simulink model "furuta_model_mabx3"  (R2023a)
settings: Solver=ode4  StartTime=0.0  StopTime=Inf  FixedStep=0.0001  RelTol=1e-3
PostLoadFcn:
  | if any(exist('dsrtsu_mdlpostloadfcn', 'file') ~= 0), dsrtsu_mdlpostloadfcn('Execute', bdroot); end
InitFcn:
  | , if any(exist('rtifpga_mdlclblib', 'file') ~= 0), rtifpga_mdlclblib('Init', bdroot); end,
  | , if any(exist('dsmpb_private', 'file') ~= 0), dsmpb_private('dsmpb_mdlclblib', 'Init', bdroot); end,
values from neighbouring files (symbols this model uses):
  N = 10    [main.m]
  nu = model.nu    [build_furuta_solver.m]    (also in furuta_model.m = 1)
  u_guess = []    [init_acados.m]    (also in main.m = u_guess.*0)
  U_max = 0.45    [build_furuta_solver.m]
  x_guess = []    [init_acados.m]    (also in main.m = x_guess.*0)
libraries: dsmpblib x7
PreSaveFcn:
  | , if any(exist('dsmpb_private', 'file') ~= 0), dsmpb_private('dsmpb_mdlclblib', 'PreSave', bdroot); end,
CloseFcn:
  | , if any(exist('dsmpb_private', 'file') ~= 0), dsmpb_private('dsmpb_mdlclblib', 'Close', bdroot); end,
settings Model: DSMPB_ID_DATA={'1',struct('BlockId','6705de95-315a-461d-bfd7-1d67e64644f6','SignalIds',{{'49302566-356f-49bf-98bb-9aa6fb4e191b','f31ab410-41a0-445c-9301-5feda3504579','b22d9c4c-e6f3-4bfe-8bb5-6e4393d82da2'}}),'2',struct('BlockId','f9af9559-7bc3-45d6-b1d0-5c923c8951f7','SignalIds',{{'640344fd-7088-4d66-828d-406be9e46a9a','f41eff98-ab4f-4f5a-b741-4dfa8486b01f','af830440-76be-4c05-a08e-eefdfbf4871e'}}),'3',struct('BlockId','0291cf52-f48d-4672-a85b-081e15b1279d','SignalIds',{{'e20d8ff1-f905-4273-8ec5-4042e75d6105'}}),'4',struct('BlockId','0211d645-065f-47f6-9582-474f3a925957','SignalIds',{{'87b883c8-a41c-4fe6-8e21-4008e8d0922c'}}),'638',struct('BlockId','b5183b78-be20-49f0-9629-cfa4d2b3c941','SignalIds',{{'6529a514-a319-41fc-97f5-7ffd89b6ed41'}}),'713',struct('BlockId','82a394dd-dc12-45ab-a2a7-927c4dc0309e','SignalIds',{{'23ea7b01-2a1b-4880-b37c-75c28e25102c'}}),'726',struct('BlockId','c77f6c66-3d30-4e59-bdfc-9087e5bcb58e','SignalIds',{{'b3d2d346-b033-4397-a923-174abd11d15c'}})}  RTICANMMDATA=struct('GeneralSetupData',struct('modelroot','C:\Users\Administrator\Furuta','generalsettings',struct('filesettings',struct('destfolder',struct('Name','RTICANMM_FILES','Check',1),'buildfolder',struct('Name','.','Check',1),'AbsDestfolder',struct('Name','C:\Users\Administrator\Furuta\RTICANMM_FILES'),'AbsBuildfolder',struct('Name','C:\Users\Administrator\Furuta'))),'options',struct('addpaths',1,'rmpaths',1,'addtrcexclusion',false,'cannavigator',struct('checkmonitoring',0),'show_usrtrc',0,'use_usrtrc',0),'advanced',struct('options',ones(1,100)),'MPSetup',{{}},'RTI',struct('Type','DSRT','Ver','4.5','Date','02-May-2021'),'modelname','Furuta_Model','block','Furuta_Model'))  DSRTSU_INTERNAL_RTIFPGA=170  Creator=Administrator  LastModifiedBy=Administrator
settings OptimizationCC: BlockReduction=off  ConditionallyExecuteInputs=off  OptimizeBlockIOStorage=off  BufferReuse=off
settings DebuggingCC: TasksWithSamePriorityMsg=none
settings HardwareCC: ProdBitPerPointer=32  ProdBitPerSizeT=32  ProdBitPerPtrDiffT=32  ProdLargestAtomicInteger=Integer  ProdWordSize=32  ProdLongLongMode=on  ProdHWDeviceType=Custom Processor->Custom
settings ModelReferenceCC: EnableParallelModelReferenceBuilds=on
settings RTWCC: Description=dSPACE Run-Time Target (for VEOS on Windows and ConfigurationDesk)  SystemTargetFile=dsrt.tlc  GenCodeOnly=on  MakeCommand=make_dsrt  TemplateMakefile=dsrt_default_tmf  RTWVerbose=off
settings RTWCC: CustomInclude=|
  | "C:\Users\Administrator\acados_neu\buildDS1403\install\include"
  | "C:\Users\Administrator\acados_neu\buildDS1403\install\include\blasfeo"
  | "C:\Users\Administrator\acados_neu\buildDS1403\install\include\blasfeo\include"
  | "C:\Users\Administrator\acados_neu\buildDS1403\install\include\acados_c"
  | "C:\Users\Administrator\acados_neu\buildDS1403\install\include\hpipm"
  | "C:\Users\Administrator\acados_neu\buildDS1403\install\include\hpipm\include"
  | "C:\Users\Administrator\acados_neu\buildDS1403\install\include\acados"
  | "C:\Users\Administrator\acados_neu\buildDS1403\install\include\acados\dense_qp"
  | "C:\Users\Administrator\acados_neu\buildDS1403\install\include\acados\ocp_nlp"
  | "C:\Users\Administrator\acados_neu\buildDS1403\install\include\acados\ocp_qp"
  | "C:\Users\Administrator\acados_neu\buildDS1403\install\include\acados\sim"
  | "C:\Users\Administrator\acados_neu\buildDS1403\install\include\acados\utils"
settings RTWCC: CustomSource=|
  | "C:\Users\Administrator\Furuta\c_generated_code\furuta_model\furuta_expl_ode_fun.c"
  | "C:\Users\Administrator\Furuta\c_generated_code\furuta_model\furuta_expl_ode_hess.c"
  | "C:\Users\Administrator\Furuta\c_generated_code\furuta_model\furuta_expl_vde_adj.c"
  | "C:\Users\Administrator\Furuta\c_generated_code\furuta_model\furuta_expl_vde_forw.c"
  | "C:\Users\Administrator\Furuta\c_generated_code\acados_solver_furuta.c"
settings RTWCC: CustomLibrary=|
  | "C:\Users\Administrator\acados_neu\buildDS1403\install\lib\libacados.a"
  | "C:\Users\Administrator\acados_neu\buildDS1403\install\lib\libblasfeo.a"
  | "C:\Users\Administrator\acados_neu\buildDS1403\install\lib\libhpipm.a"
settings STFCustomTargetCC: ParMdlRefBuildCompliant=on  ConcurrentExecutionCompliant=off  GRTInterface=off  UseToolchainInfoCompliant=off  SystemTargetFile=dsrt.tlc
settings GRTTargetCC: CompOptLevelCompliant=off  ConcurrentExecutionCompliant=off  CombineOutputUpdateFcns=off  MatFileLogging=off  CPPClassGenCompliant=off  UseToolchainInfoCompliant=off

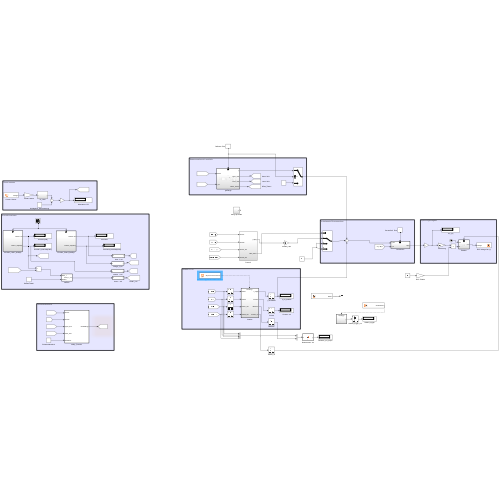
[thumbnail: Simulink's stored preview of the top-level diagram]
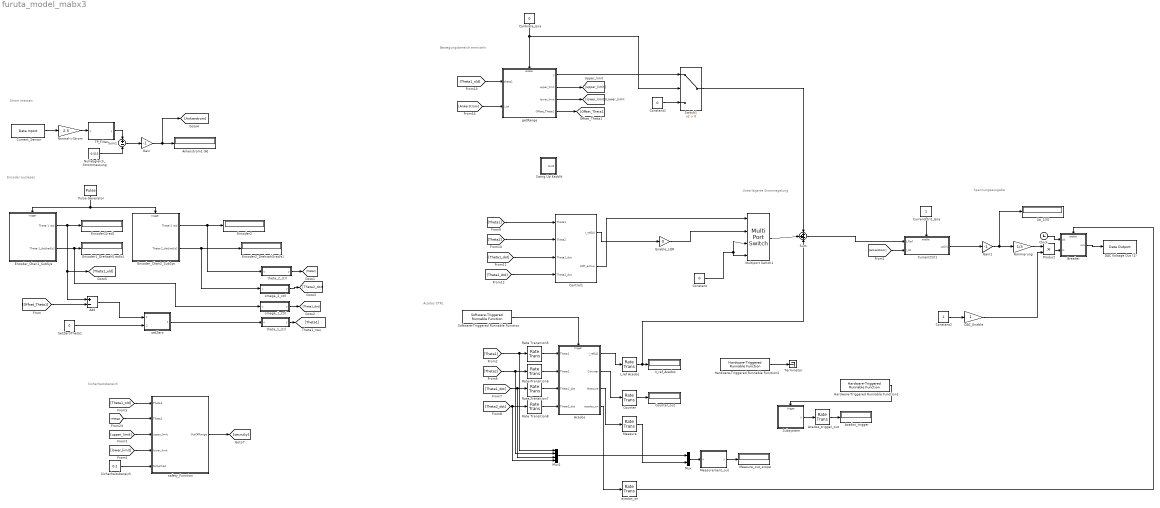
== system furuta_model_mabx3 ==
  note: Spannungsausgabe
  note: Sicherheitsbereich
  note: Bewegungsbereich ermitteln
  note: Encoder auslesen
  note: Strom messen
  note: Unterlagerte Stromregelung
  note: Acados CTRL
  Acados : Subsystem
  Acados_trigger : Display
  Acados_trigger_out : RateTransition  Deterministic=off
  Add : Sum  Inputs=+-
  Ankerstrom1 [A] : Display
  Breaker : Subsystem
  Calibrate_Ena : Constant  Value=0
  Clock : Clock
  Constant : Constant  Value=0
  Constant1 : Constant  Value=0
  Constant2 : Constant
  Control1 : Subsystem
  Counter : RateTransition  Deterministic=off
  Counter_out : Display
  CurrentCtrl1 : Subsystem
  CurrentCtrl1_Ena : Constant
  Current_Sensor : dsmpblib/Data Inport  Priority=10000
      settings: SourceProductName=dSPACE Model Interface Blockset
  DAC Voltage Out (1) : dsmpblib/Data Outport  Priority=-10000
      settings: SourceProductName=dSPACE Model Interface Blockset
  DAC_Enable : Gain
  Enable_LQR : Gain  Gain=0
  Encoder1[rad] : Display
  Encoder1_Drehzahl[rad/s] : Display
  Encoder2 : Display
  Encoder2_Drehzahl[rad/s] : Display
  Encoder_Chan1_SubSys : Subsystem
  Encoder_Chan2_SubSys : Subsystem
  Gain : Gain  Gain=-1
  Gain1 : Gain  Gain=-1
  Hardware-Triggered Runnable Function1 : dsmpblib/Hardware-Triggered Runnable Function
      settings: SourceProductName=dSPACE Model Interface Blockset
  Hardware-Triggered Runnable Function2 : dsmpblib/Hardware-Triggered Runnable Function
      settings: SourceProductName=dSPACE Model Interface Blockset
  II_ref_Acados : Display
  I_ref Acados : RateTransition  Deterministic=off
  Measure : RateTransition  Deterministic=off
  Measure_out_scope : Display
  Measurement_out : MATLAB Function  TreatAsAtomicUnit=on
  Multiport Switch1 : MultiPortSwitch  Inputs=2  DataPortForDefault=Additional data port  SaturateOnIntegerOverflow=off  InputSameDT=off
  Mux : Mux  Inputs=2
  Mux1 : Mux
  Normal->Strom : Gain  Gain=2.5
  Normierung : Gain  Gain=1/3
  Nullabgleich_Strommessung : Constant  Value=-0.015
  Product : Product
  Pulse Generator : DiscretePulseGenerator  PulseType=Time based  Period=0.001  PulseWidth=50
  Rate Transition{5..8} (4 alike) : RateTransition  Deterministic=off
  SetZeroTheta1 : Constant  Value=0
  Sicherheitsbereich : Constant  Value=0.2
  Software-Triggered Runnable Function : dsmpblib/Software-Triggered Runnable Function
      settings: SourceProductName=dSPACE Model Interface Blockset
  Subsystem : Subsystem
  Sum : Sum  Inputs=+++
  Sum1 : Sum  Inputs=+-
  Swing Up Kaddik : Subsystem
  Switch1 : Switch  Criteria=u2 > Threshold  SaturateOnIntegerOverflow=off  InputSameDT=off
  TP_Filter : Subsystem
  Terminator : Terminator
  Ua_1[V] : Display
  acados_on : RateTransition  Deterministic=off
  getRange : Subsystem
  omega_1_ctrl : MATLAB Function  TreatAsAtomicUnit=on
  omega_2_ctrl : MATLAB Function  TreatAsAtomicUnit=on
  safety_Function : MATLAB Function  TreatAsAtomicUnit=on
  setZero : MATLAB Function  TreatAsAtomicUnit=on
  theta_1_ctrl : MATLAB Function  TreatAsAtomicUnit=on
  theta_2_ctrl : MATLAB Function  TreatAsAtomicUnit=on
  wires:
  Constant1/1 -> Switch1/3
  getRange/1(y) -> Switch1/1
  [Theta1_old] -> safety_Function/1(Theta1)
  Sum/1 -> CurrentCtrl1/1(I_Ref)
  getRange/3(lower_limit) -> [lower_limit]
  Current_Sensor/1 -> Normal->Strom/1
  Pulse Generator/1 -> Encoder_Chan2_SubSys/Trigger, Encoder_Chan1_SubSys/Trigger
  Calibrate_Ena/1 -> Switch1/2, getRange/Enable
  Gain1/1 -> Normierung/1, Ua_1[V]/1
  Sum1/1 -> Gain/1
  [lower_limit] -> safety_Function/4(lower_limit)
  Gain/1 -> Ankerstrom1 [A]/1, [Ankerstrom]
  Sicherheitsbereich/1 -> safety_Function/5(Sicherheit)
  [upper_limit] -> safety_Function/3(upper_limit)
  [Ankerstrom] -> CurrentCtrl1/2(I_Ist)
  [Theta2] -> safety_Function/2(Theta2)
  TP_Filter/1(y) -> Sum1/1
  Normierung/1 -> Product/1
  [Ankerstrom] -> getRange/2(i_ist)
  CurrentCtrl1_Ena/1 -> CurrentCtrl1/Enable
  Nullabgleich_Strommessung/1 -> Sum1/2
  CurrentCtrl1/1(ua[V]) -> Gain1/1
  [Theta1_old] -> getRange/1(theta1)
  safety_Function/1(OutOfRange) -> [secruity]
  getRange/4(Offset_Theta1) -> [Offset_Theta1]
  Encoder_Chan1_SubSys/1(Theta-1 rad) -> [Theta1_old], Add/1, Encoder1[rad]/1
  getRange/2(upper_limit) -> [upper_limit]
  Normal->Strom/1 -> TP_Filter/1(u)
  [Offset_Theta1] -> Add/2
  Switch1/1 -> Sum/1
  Rate Transition5/1 -> Acados/1(Theta1)
  Acados/1(I_ref[A]) -> I_ref Acados/1
  Rate Transition8/1 -> Acados/4(Theta2_dot)
  Rate Transition7/1 -> Acados/3(Theta1_dot)
  Rate Transition6/1 -> Acados/2(Theta2)
  [Theta2] -> Mux1/2, Rate Transition6/1
  [Theta1_dot] -> Mux1/3, Rate Transition7/1
  [Theta2_dot] -> Mux1/4, Rate Transition8/1
  [Theta1] -> Control1/1(Theta1)
  [Theta2] -> Control1/2(Theta2)
  [Theta1_dot] -> Control1/3(Theta1_dot)
  [Theta2_dot] -> Control1/4(Theta2_dot)
  Control1/1(I_ref[A]) -> Enable_LQR/1
  I_ref Acados/1 -> Sum/3, II_ref_Acados/1
  Breaker/1(out) -> DAC Voltage Out (1)/1
  theta_2_ctrl/1(y) -> [Theta2]
  theta_1_ctrl/1(y) -> [Theta1]
  omega_1_ctrl/1(y) -> [Theta1_dot]
  omega_2_ctrl/1(y) -> [Theta2_dot]
  Software-Triggered Runnable Function/1 -> Acados/Trigger
  Acados/2(Counter) -> Counter/1
  Counter/1 -> Counter_out/1
  Enable_LQR/1 -> Multiport Switch1/2
  Add/1 -> setZero/1(theta_1)
  SetZeroTheta1/1 -> setZero/2(setZero)
  Control1/2(LQR_active) -> Multiport Switch1/1
  Multiport Switch1/1 -> Sum/2
  Constant/1 -> Multiport Switch1/3, Multiport Switch1/4
  [Theta1] -> Mux1/1, Rate Transition5/1
  Encoder_Chan2_SubSys/1(Theta-2 rad) -> theta_2_ctrl/1(u), Encoder2/1
  Encoder_Chan2_SubSys/2(Theta-2_dot[rad/s]) -> omega_2_ctrl/1(u), Encoder2_Drehzahl[rad/s]/1
  Encoder_Chan1_SubSys/2(Theta-1_dot[rad/s]) -> omega_1_ctrl/1(u), Encoder1_Drehzahl[rad/s]/1
  setZero/1(theta_1_out) -> theta_1_ctrl/1(u)
  Acados/3(Measure) -> Measure/1
  Measure/1 -> Mux/2
  Hardware-Triggered Runnable Function1/1 -> Subsystem/Trigger
  Subsystem/1(y) -> Acados_trigger_out/1
  Acados_trigger_out/1 -> Acados_trigger/1
  Hardware-Triggered Runnable Function2/1 -> Terminator/1
  Mux/1 -> Measurement_out/1(u)
  Mux1/1 -> Mux/1
  Measurement_out/1(y) -> Measure_out_scope/1
  Constant2/1 -> DAC_Enable/1
  DAC_Enable/1 -> Product/2
  Product/1 -> Breaker/2(in)
  Clock/1 -> Breaker/1(clk)
  Acados/4(acados_on) -> acados_on/1
  acados_on/1 -> Breaker/Enable

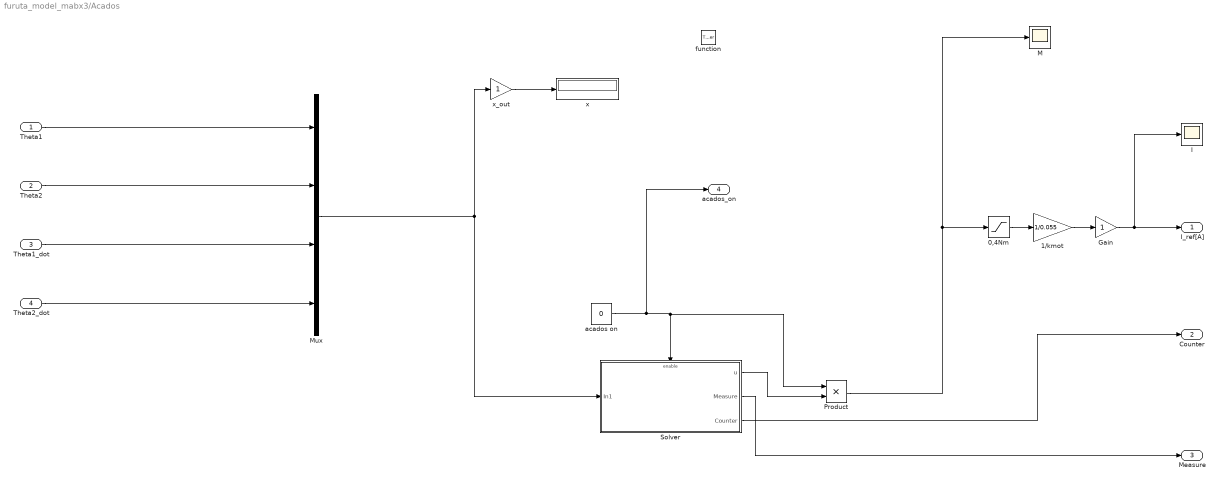
== system furuta_model_mabx3/Acados ==
  Theta1 : Inport
  Theta2 : Inport  Port=2
  Theta1_dot : Inport  Port=3
  Theta2_dot : Inport  Port=4
  function : TriggerPort  TriggerType=function-call  VariantControl=Variant
  0,4Nm : Saturate  UpperLimit=0.4  LowerLimit=-0.4
  1/kmot : Gain  Gain=1/0.055
  Gain : Gain
  I : Scope
  M : Scope
  Mux : Mux
  Product : Product
  Solver : Subsystem
  acados on : Constant  Value=0
  x : Display
  x_out : Gain
  I_ref[A] : Outport  OutputWhenDisabled=reset  InitialOutput=0  VectorParamsAs1DForOutWhenUnconnected=off
  Counter : Outport  Port=2  OutputWhenDisabled=reset  InitialOutput=0  VectorParamsAs1DForOutWhenUnconnected=off
  Measure : Outport  Port=3  OutputWhenDisabled=reset  InitialOutput=0  VectorParamsAs1DForOutWhenUnconnected=off
  acados_on : Outport  Port=4  OutputWhenDisabled=reset  InitialOutput=0  VectorParamsAs1DForOutWhenUnconnected=off
  wires:
  1/kmot/1 -> Gain/1
  Theta2/1 -> Mux/2
  Theta1/1 -> Mux/1
  0,4Nm/1 -> 1/kmot/1
  Theta2_dot/1 -> Mux/4
  Theta1_dot/1 -> Mux/3
  Gain/1 -> I/1, I_ref[A]/1
  x_out/1 -> x/1
  Mux/1 -> x_out/1, Solver/1(In1)
  Product/1 -> 0,4Nm/1, M/1
  acados on/1 -> acados_on/1, Product/1, Solver/Enable
  Solver/1(u) -> Product/2
  Solver/2(Measure) -> Measure/1
  Solver/3(Counter) -> Counter/1

== system furuta_model_mabx3/Breaker ==
  clk : Inport
  in : Inport  Port=2
  Enable : EnablePort
  MATLAB Function : MATLAB Function  TreatAsAtomicUnit=on
  out : Outport
  wires:
  MATLAB Function/1(out) -> out/1
  in/1 -> MATLAB Function/2(in)
  clk/1 -> MATLAB Function/1(clk)

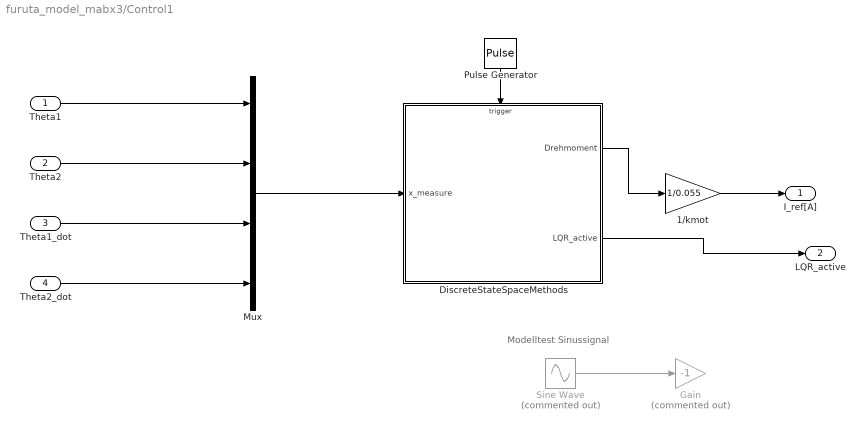
== system furuta_model_mabx3/Control1 ==
  note: Modelltest Sinussignal
  Theta1 : Inport
  Theta2 : Inport  Port=2
  Theta1_dot : Inport  Port=3
  Theta2_dot : Inport  Port=4
  1/kmot : Gain  Gain=1/0.055
  DiscreteStateSpaceMethods : Subsystem
  Gain : Gain  Commented=on  Gain=-1
  Mux : Mux
  Pulse Generator : DiscretePulseGenerator  PulseType=Time based  Period=0.001  PulseWidth=50
  Sine Wave : Sin  Commented=on  Amplitude=1.22  Bias=0.3  Frequency=0.8  SampleTime=0
  I_ref[A] : Outport  OutputWhenDisabled=reset  InitialOutput=0  VectorParamsAs1DForOutWhenUnconnected=off
  LQR_active : Outport  Port=2  OutputWhenDisabled=reset  InitialOutput=0  VectorParamsAs1DForOutWhenUnconnected=off
  wires:
  DiscreteStateSpaceMethods/1(Drehmoment) -> 1/kmot/1
  Pulse Generator/1 -> DiscreteStateSpaceMethods/Trigger
  Theta1/1 -> Mux/1
  Theta2/1 -> Mux/2
  Theta1_dot/1 -> Mux/3
  Theta2_dot/1 -> Mux/4
  Mux/1 -> DiscreteStateSpaceMethods/1(x_measure)
  Sine Wave/1 -> Gain/1
  1/kmot/1 -> I_ref[A]/1
  DiscreteStateSpaceMethods/2(LQR_active) -> LQR_active/1

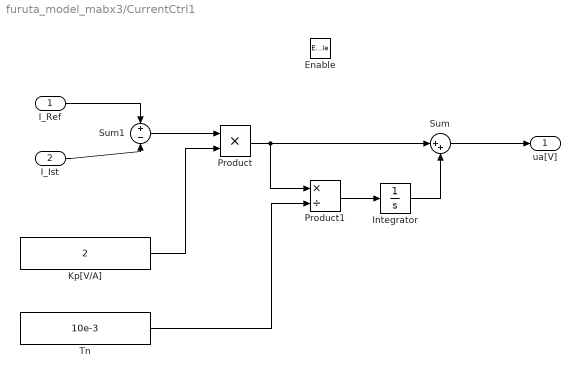
== system furuta_model_mabx3/CurrentCtrl1 ==
  I_Ref : Inport
  I_Ist : Inport  Port=2
  Enable : EnablePort  StatesWhenEnabling=reset
  Integrator : Integrator  LimitOutput=on  UpperSaturationLimit=10  LowerSaturationLimit=-10
  Kp[V/A] : Constant  Value=2
  Product : Product  RndMeth=Zero
  Product1 : Product  Inputs=*/  RndMeth=Zero
  Sum : Sum  Inputs=|++
  Sum1 : Sum  Inputs=+-
  Tn : Constant  Value=10e-3
  ua[V] : Outport  OutputWhenDisabled=reset  InitialOutput=0  VectorParamsAs1DForOutWhenUnconnected=off
  wires:
  I_Ref/1 -> Sum1/1
  I_Ist/1 -> Sum1/2
  Sum1/1 -> Product/1
  Kp[V/A]/1 -> Product/2
  Product/1 -> Sum/1, Product1/1
  Integrator/1 -> Sum/2
  Product1/1 -> Integrator/1
  Tn/1 -> Product1/2
  Sum/1 -> ua[V]/1

== system furuta_model_mabx3/Encoder_Chan1_SubSys ==
  Trigger : TriggerPort  VariantControl=(inherit)
  CONST1 : Constant  Value=pi/180*2
  DT1 : Display
  DT1 Transfer Fcn : DiscreteTransferFcn  Numerator=[50, -50]  Denominator=[1, -0.9512]
  Enc position : Display
  Enc_1 : dsmpblib/Data Inport  Priority=10000
      settings: SourceProductName=dSPACE Model Interface Blockset
  Product3 : Product  RndMeth=Zero
  Theta-1 rad : Outport  VectorParamsAs1DForOutWhenUnconnected=off
  Theta-1_dot[rad/s] : Outport  Port=2  VectorParamsAs1DForOutWhenUnconnected=off
  wires:
  Enc_1/2 -> Product3/1, Enc position/1
  CONST1/1 -> Product3/2
  DT1 Transfer Fcn/1 -> Theta-1_dot[rad/s]/1, DT1/1
  Product3/1 -> Theta-1 rad/1, DT1 Transfer Fcn/1

== system furuta_model_mabx3/Encoder_Chan2_SubSys ==
  Trigger : TriggerPort  VariantControl=(inherit)
  CONST1 : Constant  Value=pi/180*2
  DT1 Transfer Fcn : DiscreteTransferFcn  Numerator=[50, -50]  Denominator=[1, -0.9512]
  Enc_2 : dsmpblib/Data Inport  Priority=10000
      settings: SourceProductName=dSPACE Model Interface Blockset
  Product3 : Product  RndMeth=Zero
  Theta-2 rad : Outport  VectorParamsAs1DForOutWhenUnconnected=off
  Theta-2_dot[rad/s] : Outport  Port=2  VectorParamsAs1DForOutWhenUnconnected=off
  wires:
  Enc_2/2 -> Product3/1
  CONST1/1 -> Product3/2
  DT1 Transfer Fcn/1 -> Theta-2_dot[rad/s]/1
  Product3/1 -> DT1 Transfer Fcn/1, Theta-2 rad/1

== system furuta_model_mabx3/Subsystem ==
  function : TriggerPort  TriggerType=function-call  VariantControl=Variant
  MATLAB Function : MATLAB Function  TreatAsAtomicUnit=on
  y : Outport
  wires:
  MATLAB Function/1(y) -> y/1

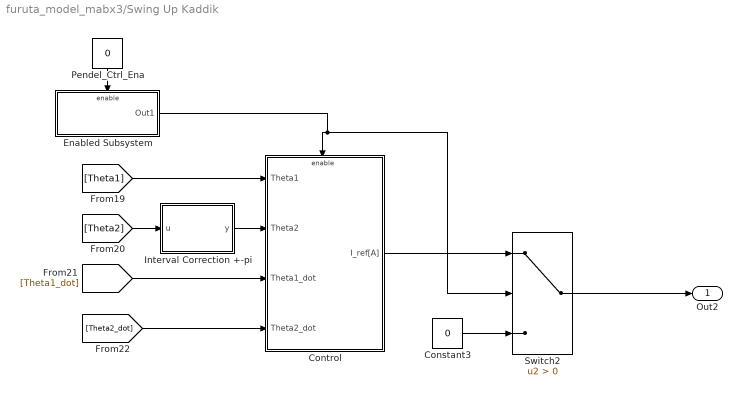
== system furuta_model_mabx3/Swing Up Kaddik ==
  Constant3 : Constant  Value=0
  Control : Subsystem
  Enabled Subsystem : Subsystem  TreatAsAtomicUnit=on
  Interval Correction +-pi : MATLAB Function  TreatAsAtomicUnit=on
  Pendel_Ctrl_Ena : Constant  Value=0
  Switch2 : Switch  Criteria=u2 > Threshold  SaturateOnIntegerOverflow=off  InputSameDT=off
  Out2 : Outport
  wires:
  Enabled Subsystem/1(Out1) -> Control/Enable, Switch2/2
  Constant3/1 -> Switch2/3
  [Theta1] -> Control/1(Theta1)
  [Theta2_dot] -> Control/4(Theta2_dot)
  [Theta1_dot] -> Control/3(Theta1_dot)
  Interval Correction +-pi/1(y) -> Control/2(Theta2)
  Control/1(I_ref[A]) -> Switch2/1
  Pendel_Ctrl_Ena/1 -> Enabled Subsystem/Enable
  [Theta2] -> Interval Correction +-pi/1(u)
  Switch2/1 -> Out2/1

== system furuta_model_mabx3/TP_Filter ==
  u : Inport
  Integrator : Integrator  UpperSaturationLimit=10  LowerSaturationLimit=-10
  Product : Product  Inputs=*/  RndMeth=Zero
  Sum1 : Sum  Inputs=+-
  ms->s : Gain  Gain=0.001
  "tau[ms}" : Constant
  y : Outport  OutputWhenDisabled=reset  InitialOutput=0  VectorParamsAs1DForOutWhenUnconnected=off
  wires:
  Integrator/1 -> y/1, Sum1/2
  "tau[ms}"/1 -> ms->s/1
  Sum1/1 -> Product/1
  u/1 -> Sum1/1
  Product/1 -> Integrator/1
  ms->s/1 -> Product/2

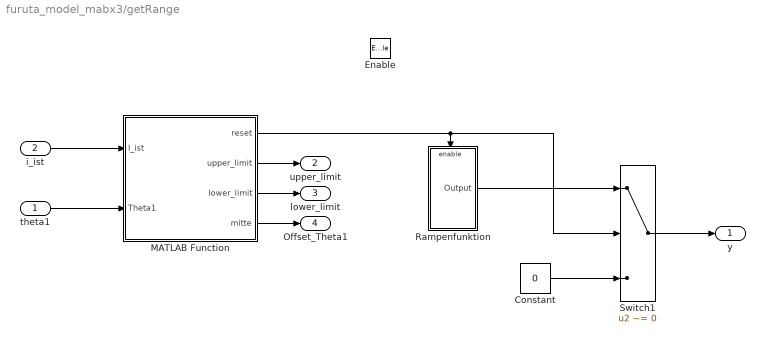
== system furuta_model_mabx3/getRange ==
  theta1 : Inport
  i_ist : Inport  Port=2
  Enable : EnablePort
  Constant : Constant  Value=0
  MATLAB Function : MATLAB Function  TreatAsAtomicUnit=on
  Rampenfunktion : Subsystem
  Switch1 : Switch  Criteria=u2 ~= 0  SaturateOnIntegerOverflow=off  InputSameDT=off
  y : Outport  OutputWhenDisabled=reset  InitialOutput=[0]
  upper_limit : Outport  Port=2
  lower_limit : Outport  Port=3
  Offset_Theta1 : Outport  Port=4
  wires:
  theta1/1 -> MATLAB Function/2(Theta1)
  i_ist/1 -> MATLAB Function/1(I_ist)
  MATLAB Function/1(reset) -> Switch1/2, Rampenfunktion/Enable
  MATLAB Function/3(lower_limit) -> lower_limit/1
  MATLAB Function/2(upper_limit) -> upper_limit/1
  Rampenfunktion/1(Output) -> Switch1/1
  Constant/1 -> Switch1/3
  Switch1/1 -> y/1
  MATLAB Function/4(mitte) -> Offset_Theta1/1

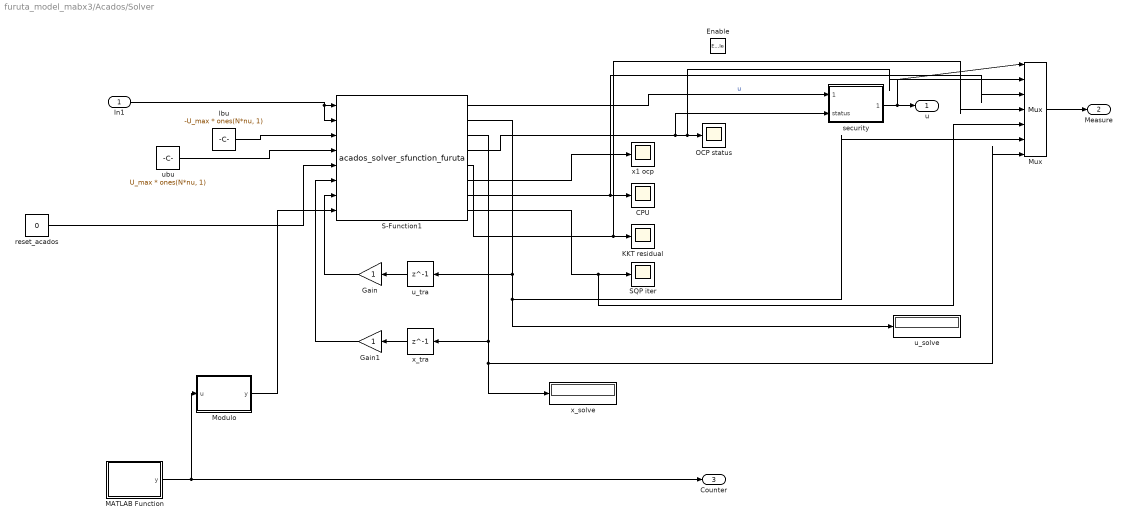
== system furuta_model_mabx3/Acados/Solver ==
  In1 : Inport
  Enable : EnablePort
  CPU : Scope
      settings: Description=status
  Gain : Gain
  Gain1 : Gain
  KKT residual : Scope
      settings: Description=status
  MATLAB Function : MATLAB Function  TreatAsAtomicUnit=on
  Modulo : MATLAB Function  TreatAsAtomicUnit=on
  Mux : Mux  Inputs=7
  OCP status : Scope
      settings: Description=status
  S-Function1 : S-Function  FunctionName=acados_solver_sfunction_furuta  SFunctionDeploymentMode=off  EnableBusSupport=off
  SQP iter : Scope
      settings: Description=status
  lbu : Constant  Value=-U_max * ones(N*nu, 1)
  reset_acados : Constant  Value=0
  security : MATLAB Function  TreatAsAtomicUnit=on
  u_solve : Display
  u_tra : Delay  DelayLength=1  InitialCondition=u_guess
  ubu : Constant  Value=U_max * ones(N*nu, 1)
  x1 ocp : Scope
      settings: Description=status
  x_solve : Display
  x_tra : Delay  DelayLength=1  InitialCondition=x_guess
  u : Outport
  Measure : Outport  Port=2
  Counter : Outport  Port=3
  wires:
  S-Function1/6 -> x1 ocp/1
  S-Function1/2 -> Mux/6, u_solve/1, u_tra/1
  In1/1 -> S-Function1/2, S-Function1/1
  S-Function1/3 -> x_tra/1, Mux/7, x_solve/1
  u_tra/1 -> Gain/1
  S-Function1/7 -> Mux/3, CPU/1
  S-Function1/5 -> Mux/4, KKT residual/1
  ubu/1 -> S-Function1/4
  lbu/1 -> S-Function1/3
  S-Function1/4 -> security/2(status), Mux/2, OCP status/1
  S-Function1/8 -> Mux/5, SQP iter/1
  S-Function1/1 -> security/1(control)  "u"
  x_tra/1 -> Gain1/1
  security/1(control_out) -> Mux/1, u/1
  Gain/1 -> S-Function1/7
  Gain1/1 -> S-Function1/6
  reset_acados/1 -> S-Function1/5
  Mux/1 -> Measure/1
  MATLAB Function/1(y) -> Modulo/1(u), Counter/1
  Modulo/1(y) -> S-Function1/8

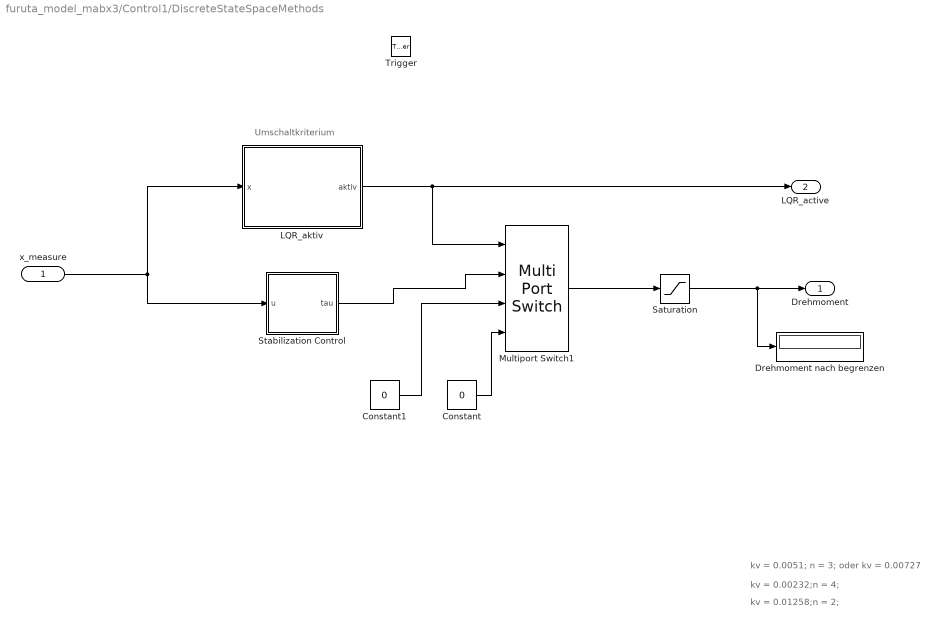
== system furuta_model_mabx3/Control1/DiscreteStateSpaceMethods ==
  note: kv = 0.00232;n = 4;
  note: kv = 0.0051; n = 3; oder kv = 0.00727
  note: Umschaltkriterium
  note: kv = 0.01258;n = 2;
  x_measure : Inport
  Trigger : TriggerPort  VariantControl=(inherit)  PortDimensions=1
  Constant : Constant  Value=0
  Constant1 : Constant  Value=0
  Drehmoment nach begrenzen : Display
  LQR_aktiv : MATLAB Function  TreatAsAtomicUnit=on
  Multiport Switch1 : MultiPortSwitch  Inputs=2  DataPortForDefault=Additional data port  SaturateOnIntegerOverflow=off  InputSameDT=off
  Saturation : Saturate  UpperLimit=0.4  LowerLimit=-0.4
  Stabilization Control : Subsystem
  Drehmoment : Outport  VectorParamsAs1DForOutWhenUnconnected=off
  LQR_active : Outport  Port=2  VectorParamsAs1DForOutWhenUnconnected=off
  wires:
  Saturation/1 -> Drehmoment nach begrenzen/1, Drehmoment/1
  LQR_aktiv/1(aktiv) -> LQR_active/1, Multiport Switch1/1
  x_measure/1 -> LQR_aktiv/1(x), Stabilization Control/1(u)
  Constant/1 -> Multiport Switch1/4
  Stabilization Control/1(tau) -> Multiport Switch1/2
  Multiport Switch1/1 -> Saturation/1
  Constant1/1 -> Multiport Switch1/3

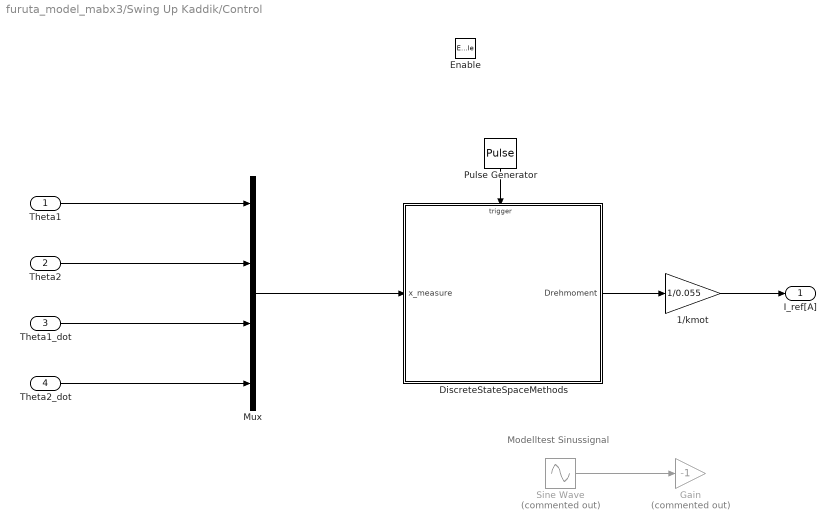
== system furuta_model_mabx3/Swing Up Kaddik/Control ==
  note: Modelltest Sinussignal
  Theta1 : Inport
  Theta2 : Inport  Port=2
  Theta1_dot : Inport  Port=3
  Theta2_dot : Inport  Port=4
  Enable : EnablePort  StatesWhenEnabling=reset
  1/kmot : Gain  Gain=1/0.055
  DiscreteStateSpaceMethods : Subsystem
  Gain : Gain  Commented=on  Gain=-1
  Mux : Mux
  Pulse Generator : DiscretePulseGenerator  PulseType=Time based  Period=0.001  PulseWidth=50
  Sine Wave : Sin  Commented=on  Amplitude=1.22  Bias=0.3  Frequency=0.8  SampleTime=0
  I_ref[A] : Outport  OutputWhenDisabled=reset  InitialOutput=0  VectorParamsAs1DForOutWhenUnconnected=off
  wires:
  DiscreteStateSpaceMethods/1(Drehmoment) -> 1/kmot/1
  Pulse Generator/1 -> DiscreteStateSpaceMethods/Trigger
  Theta1/1 -> Mux/1
  Theta2/1 -> Mux/2
  Theta1_dot/1 -> Mux/3
  Theta2_dot/1 -> Mux/4
  Mux/1 -> DiscreteStateSpaceMethods/1(x_measure)
  Sine Wave/1 -> Gain/1
  1/kmot/1 -> I_ref[A]/1

== system furuta_model_mabx3/Swing Up Kaddik/Enabled Subsystem ==
  Enable : EnablePort  StatesWhenEnabling=reset
  Pulse Generator1 : DiscretePulseGenerator  PulseType=Time based  Period=20  PulseWidth=80
  Out1 : Outport
  wires:
  Pulse Generator1/1 -> Out1/1

== system furuta_model_mabx3/getRange/Rampenfunktion ==
  Enable : EnablePort  StatesWhenEnabling=reset
  Integrator1 : Integrator  InitialCondition=0.5
  Step1 : Step  Time=0  After=0.15  SampleTime=0
  Output : Outport
  wires:
  Integrator1/1 -> Output/1
  Step1/1 -> Integrator1/1

== system furuta_model_mabx3/Control1/DiscreteStateSpaceMethods/Stabilization Control ==
  u : Inport
  Add : Sum  Inputs=++++
  Demux : Demux
  LQR_Controller : MATLAB Function  TreatAsAtomicUnit=on
  k1 : Gain  Gain=0.1
  k2 : Gain  Gain=-1.3582
  k3 : Gain  Gain=0.0544
  k4 : Gain  Gain=-0.138
  tau : Outport
  wires:
  LQR_Controller/1(drehmoment_soll) -> tau/1
  u/1 -> LQR_Controller/1(x_measure)
  Demux/1 -> k1/1
  k3/1 -> Add/3
  k2/1 -> Add/2
  Demux/4 -> k4/1
  k1/1 -> Add/1
  Demux/3 -> k3/1
  Demux/2 -> k2/1
  k4/1 -> Add/4

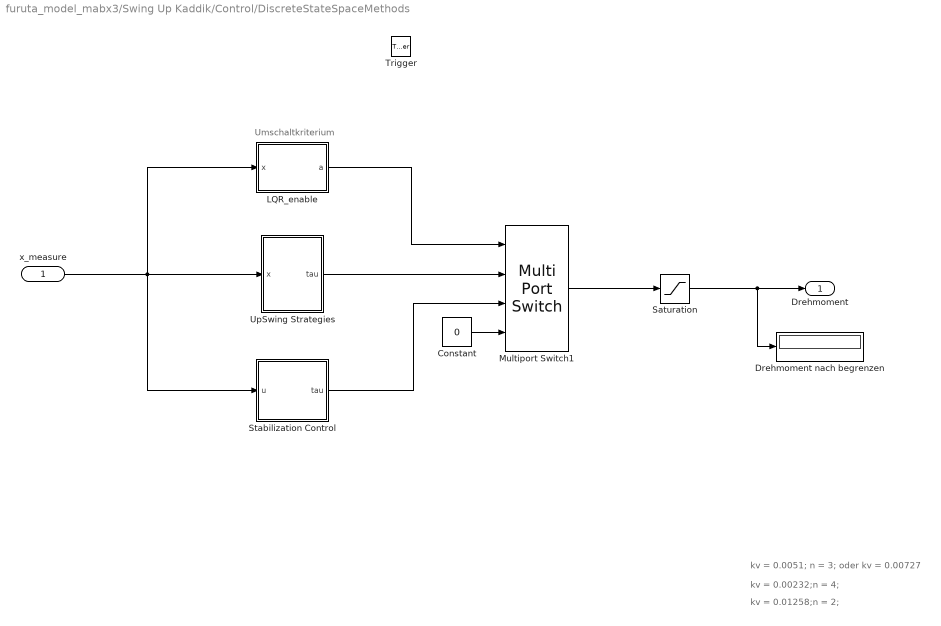
== system furuta_model_mabx3/Swing Up Kaddik/Control/DiscreteStateSpaceMethods ==
  note: kv = 0.00232;n = 4;
  note: kv = 0.0051; n = 3; oder kv = 0.00727
  note: Umschaltkriterium
  note: kv = 0.01258;n = 2;
  x_measure : Inport
  Trigger : TriggerPort  VariantControl=(inherit)  PortDimensions=1
  Constant : Constant  Value=0
  Drehmoment nach begrenzen : Display
  LQR_enable : MATLAB Function  TreatAsAtomicUnit=on
  Multiport Switch1 : MultiPortSwitch  Inputs=2  DataPortForDefault=Additional data port  SaturateOnIntegerOverflow=off  InputSameDT=off
  Saturation : Saturate  UpperLimit=0.4  LowerLimit=-0.4
  Stabilization Control : Subsystem
  UpSwing Strategies : Subsystem
  Drehmoment : Outport  VectorParamsAs1DForOutWhenUnconnected=off
  wires:
  Saturation/1 -> Drehmoment nach begrenzen/1, Drehmoment/1
  LQR_enable/1(a) -> Multiport Switch1/1
  x_measure/1 -> LQR_enable/1(x), Stabilization Control/1(u), UpSwing Strategies/1(x)
  Constant/1 -> Multiport Switch1/4
  UpSwing Strategies/1(tau) -> Multiport Switch1/2
  Stabilization Control/1(tau) -> Multiport Switch1/3
  Multiport Switch1/1 -> Saturation/1

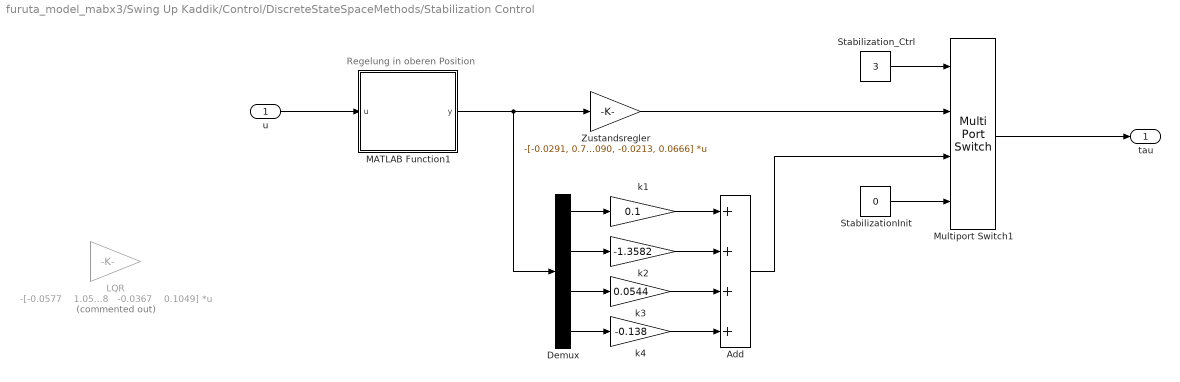
== system furuta_model_mabx3/Swing Up Kaddik/Control/DiscreteStateSpaceMethods/Stabilization Control ==
  note: Regelung in oberen Position
  u : Inport
  Add : Sum  Inputs=++++
  Demux : Demux
  LQR : Gain  Commented=on  Gain="-[-0.0577    1.0578   -0.0367    0.1049]"  Multiplication=Matrix(K*u) (u vector)
  MATLAB Function1 : MATLAB Function  TreatAsAtomicUnit=on
  Multiport Switch1 : MultiPortSwitch  Inputs=2  DataPortForDefault=Additional data port  SaturateOnIntegerOverflow=off  InputSameDT=off
  StabilizationInit : Constant  Value=0
  Stabilization_Ctrl : Constant  Value=3
  Zustandsregler : Gain  Gain=-[-0.0291, 0.7090, -0.0213, 0.0666]  Multiplication=Matrix(K*u) (u vector)
  k1 : Gain  Gain=0.1
  k2 : Gain  Gain=-1.3582
  k3 : Gain  Gain=0.0544
  k4 : Gain  Gain=-0.138
  tau : Outport
  wires:
  u/1 -> MATLAB Function1/1(u)
  StabilizationInit/1 -> Multiport Switch1/4
  Multiport Switch1/1 -> tau/1
  Add/1 -> Multiport Switch1/3
  Stabilization_Ctrl/1 -> Multiport Switch1/1
  Zustandsregler/1 -> Multiport Switch1/2
  MATLAB Function1/1(y) -> Demux/1, Zustandsregler/1
  Demux/1 -> k1/1
  k3/1 -> Add/3
  k2/1 -> Add/2
  Demux/4 -> k4/1
  k1/1 -> Add/1
  Demux/3 -> k3/1
  Demux/2 -> k2/1
  k4/1 -> Add/4

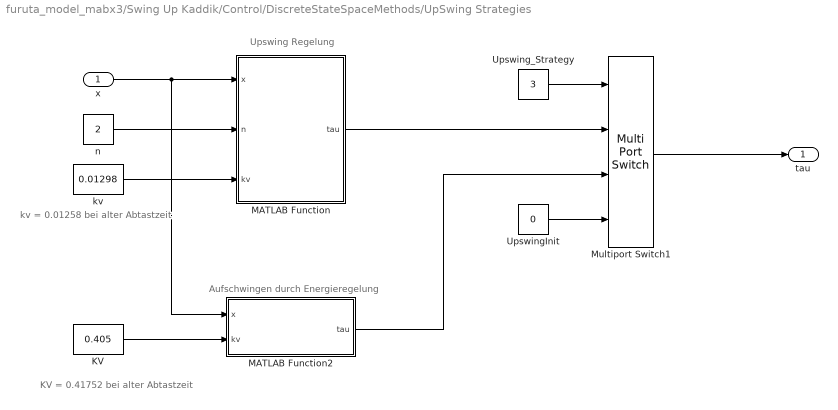
== system furuta_model_mabx3/Swing Up Kaddik/Control/DiscreteStateSpaceMethods/UpSwing Strategies ==
  note: kv = 0.01258 bei alter Abtastzeit
  note: KV = 0.41752 bei alter Abtastzeit
  note: Upswing Regelung
  note: Aufschwingen durch Energieregelung
  x : Inport
  KV : Constant  Value=0.405
  MATLAB Function : MATLAB Function  TreatAsAtomicUnit=on
  MATLAB Function2 : MATLAB Function  TreatAsAtomicUnit=on
  Multiport Switch1 : MultiPortSwitch  Inputs=2  DataPortForDefault=Additional data port  SaturateOnIntegerOverflow=off  InputSameDT=off
  UpswingInit : Constant  Value=0
  Upswing_Strategy : Constant  Value=3
  kv : Constant  Value=0.01298
  n : Constant  Value=2
  tau : Outport
  wires:
  x/1 -> MATLAB Function/1(x), MATLAB Function2/1(x)
  kv/1 -> MATLAB Function/3(kv)
  MATLAB Function/1(tau) -> Multiport Switch1/2
  n/1 -> MATLAB Function/2(n)
  KV/1 -> MATLAB Function2/2(kv)
  Upswing_Strategy/1 -> Multiport Switch1/1
  MATLAB Function2/1(tau) -> Multiport Switch1/3
  Multiport Switch1/1 -> tau/1
  UpswingInit/1 -> Multiport Switch1/4

== matlab function furuta_model_mabx3/Acados/Solver/MATLAB Function ==
  data: y output
function y = fcn()
%#codegen

persistent zahl
if isempty(zahl)
    zahl=0;
else
    zahl=zahl+1;
end
y = zahl;

== matlab function furuta_model_mabx3/setZero ==
  data: theta_1 input; theta_1_out output; setZero input
function theta_1_out = fcn(theta_1,setZero)
%#codegen
persistent offset

theta_1_out=theta_1;

if setZero==1 && isempty(offset)
    offset = theta_1;
end
if ~isempty(offset)
    theta_1_out = theta_1-offset;
end

== matlab function furuta_model_mabx3/Acados/Solver/security ==
  data: control input; control_out output; status input
function control_out = fcn(control,status)
%#codegen
control_out=0;
if status~=4
control_out = control;
end

== matlab function furuta_model_mabx3/Subsystem/MATLAB Function ==
  data: y output
function y = fcn()
%#codegen

persistent zahl
if isempty(zahl)
    zahl=0;
else
    zahl=zahl+1;
end
y = zahl;

== matlab function furuta_model_mabx3/Acados/Solver/Modulo ==
  data: u input; y output
function y = fcn(u)
%#codegen

y=mod(u,2)+1;
y=0;

== matlab function furuta_model_mabx3/Measurement_out ==
  data: u input; y output
function y = fcn(u)
%#codegen

y = u;

== matlab function furuta_model_mabx3/Breaker/MATLAB Function ==
  data: clk input; out output; in input
function out = fcn(clk,in)
%#codegen
t_min_1 = 0.2;%0.2;
t_max_1 = 0.3;%0.3;
t_min_2 = 0.6;%0.6;
t_max_2 = 0.8;%1;

persistent t_start
if isempty(t_start)
t_start=clk;
end
t=clk-t_start;
if (t<t_max_1 && t>t_min_1) ||  (t<t_max_2 && t>t_min_2)
    out=0;
else
    out=in;
end

== matlab function furuta_model_mabx3/Swing Up Kaddik/Control/DiscreteStateSpaceMethods/Stabilization Control/MATLAB Function1 ==
  data: u input; y output
function y = fcn(u)
% Ausgangsvektor erstellen
y = zeros(4,1);

% Werte auf ein -pi +pi kürzen
for i = 1:2
    vielfache = u(i)/pi;
    vorkomma = double(int8(vielfache+(sign(vielfache)*0.5*-1)));
    gerade = mod(vorkomma,2);
    rest = mod(vielfache,vorkomma);

    % wenn gerade
    if gerade == 0
        y(i) = rest*pi;
    % sonst ungerade
    else
        % positiv
        if vorkomma > 0
            y(i) = (pi-(rest*pi))*-1;
        % negativ
        elseif vorkomma < 0
            y(i) = (pi-abs(rest*pi));
        % null
        else
            y(i) = 0;
        end
    end
end
y(3) = u(3);
y(4) = u(4);

% Wenn in der linken hälfte Arbeitspunkt addieren
if y(2) < 0
    y(2) = y(2) + pi;
% sonst abziehen
else
    y(2) = y(2) - pi;
end

== matlab function furuta_model_mabx3/Swing Up Kaddik/Control/DiscreteStateSpaceMethods/LQR_enable ==
  settings: updateMethod=DISCRETE
  data: x input; a output
function a = fcn(x)

% Theta1 = x(1);
theta2 = x(2);
% Theta1_dot = x(3);
theta2_dt = x(4);

persistent st;
if isempty(st)
    st = 1;
end

max_velocity = 5;
max_angle = 2.9;


if (theta2 > max_angle || theta2 < -max_angle) && (theta2_dt < max_velocity && theta2_dt > -max_velocity)
    st = 2;
end
if st == 2 && (theta2 < max_angle-0.5 && theta2 > -max_angle+0.5)
    st = 3;
end

a = st;

% if st == 0
%     tau1 = upswing(theta2, theta2_dt);
% elseif st == 1
%     tau1 = PD(theta2);
% else
%     tau1 = 100;
% end

== matlab function furuta_model_mabx3/Swing Up Kaddik/Control/DiscreteStateSpaceMethods/UpSwing Strategies/MATLAB Function2 ==
  data: x input; tau output; kv input
function tau = fcn(x, kv)

% Theta1 = x(1);
theta2 = x(2);
% Theta1_dot = x(3);
theta2_dt = x(4);

% Parameter deklarieren
L1 = 0.1035; % 103.5mm
L2 = 0.173; % 173mm

% l1 nicht angegeben
l2 = 0.0955; % 92.1mm

% m1 nicht angegeben
m2 = 0.192; % 199g

% J1 nicht angegeben
J2 = 7.653e-04; % 765.3 kg/mm^2

g = 9.81;

% gesamte Trägheitsmoment von Arm 1 um den Drehpunkt
J1_ges = 5.3875e-04 + 0.75e-04; % J1 + m1*l1^2;
% gesamte Trägheitsmoment von Arm 2 um den Drehpunkt
J2_ges = J2 + m2*l2^2;
% Gesamtträgheitsmoment am Motor
J0 = J1_ges + m2*L1^2;

% nicht angegeben
b1 = 27*10^(-4); % Dämpfung von den Motorlagern
%b1 = 10;
k = 0.098;
b2 = 2*k*J2_ges; % Dämpfung der Bolzenkupplung zwischen Arm 1 und Arm 

% Frequenz der kleinen Schwingungen des Pendels
w0 = sqrt(m2*g*l2/J2);

% Aktuelle Energie berechnen
E = 0.5*J2*theta2_dt^2+m2*g*l2*(1-cos(theta2));
% Energie an der oberen Position
E0 = 2*m2*g*l2;

% Reglerstruktur
% kv = 1.1;
% kv = 2.9;
% kv = 4.4;
lowersat = -5;
uppersat = 5;
s = sign(theta2_dt*cos(theta2));
if s == 0
    s = 1;
end

persistent st;
if isempty(st)
    st = 1;
    s = 1;
end

tau = min(uppersat, max(lowersat, kv*(E-E0)))*s;

== matlab function furuta_model_mabx3/safety_Function ==
  data: Theta1 input; OutOfRange output; Theta2 input; upper_limit input; lower_limit input; Sicherheit input
function OutOfRange = fcn(Theta1, Theta2, upper_limit, lower_limit, Sicherheit)

% Wenn Motorachse an Stopper kommt abschalten
if Theta1 > upper_limit-Sicherheit
    OutOfRange = 1;
elseif Theta1 < lower_limit+Sicherheit
    OutOfRange = 1;
% Wenn Pendel überschlägt abschalten
elseif Theta2 > 1.3*pi || Theta2 < -1.3*pi
    OutOfRange = 1;
% Sonst laufen lassen
else
    OutOfRange = 0;
end

== matlab function furuta_model_mabx3/getRange/MATLAB Function ==
  settings: updateMethod=DISCRETE
  data: I_ist input; Theta1 input; reset output; upper_limit output; lower_limit output; mitte output
function [reset, upper_limit, lower_limit, mitte]= fcn(I_ist, Theta1)
% Durch Messung bekannt, dass Stopper 60° groß ist
% Somit 300° Bewegungsradius ca. 5.2490 rad

% Variablen deklarieren
persistent status
persistent lower
persistent upper

% Variablen beim Start einmalig deklarieren
if isempty(status)
    status = 1;
    lower = -2*pi;
    upper = 2*pi;
end

% Wenn noch kein Anschlag gefunden worden ist
if status == 1
    reset = 1;  % Rampenfunktion triggern
    mitte = 0;  % Mitte bzw Offset deklarieren
    
    % Wenn Anschlag in negativer Richtung erreicht
    if  I_ist > 2
        upper = Theta1;         % unteres Ende merken
        lower = upper - 5.2490; % oberes Ende durch addieren von 300°
        reset = 0;              % Rampenfunktion nicht mehr triggern
        status = 2;             % Status wechseln
    end
% Wenn Bewegungsbereich schon bekannt
else
    reset = 0;                  % Rampenfunktion weiterhin aus
    mitte = (lower+upper)/2;    % Mittelpunkt berechnen
end

% Ausgangsvariablen definieren
upper_limit = upper;
lower_limit = lower;

== matlab function furuta_model_mabx3/Swing Up Kaddik/Control/DiscreteStateSpaceMethods/UpSwing Strategies/MATLAB Function ==
  data: x input; n input; tau output; kv input
function tau = fcn(x,n,kv)

% Theta1 = x(1);
theta2 = x(2);
% Theta1_dot = x(3);
theta2_dt = x(4);

%kv = 0.0051;
%n = 3;
s = -sign(theta2_dt*cos(theta2));
if s == 0
    s = 1;
end

persistent st;
if isempty(st)
    st = 1;
    s = -1;
end

tau = kv*abs((abs(theta2)-pi)^n)*s;

== matlab function furuta_model_mabx3/Swing Up Kaddik/Interval Correction +-pi ==
  data: u input; y output
function y = fcn(u)

y=u;
while abs(y)>pi
    if sign(y)>0
        y=y-2*pi;
    else
        y=y+2*pi;
    end
end

== matlab function furuta_model_mabx3/theta_1_ctrl ==
  data: u input; y output
function y = fcn(u)
%#codegen

y = u;

== matlab function furuta_model_mabx3/theta_2_ctrl ==
  data: u input; y output
function y = fcn(u)
%#codegen

y = u-1*pi;

== matlab function furuta_model_mabx3/omega_1_ctrl ==
  data: u input; y output
function y = fcn(u)
%#codegen

y = u;

== matlab function furuta_model_mabx3/omega_2_ctrl ==
  data: u input; y output
function y = fcn(u)
%#codegen

y = u;

== matlab function furuta_model_mabx3/Control1/DiscreteStateSpaceMethods/Stabilization Control/LQR_Controller ==
  data: x_measure input; drehmoment_soll output
function drehmoment_soll = fcn(x_measure)

% Inputs auswerten
    x_tilde    = zeros(4,1);
    x_tilde(1) = x_measure(1); % 0 vorne
    x_tilde(2) = x_measure(2);
    x_tilde(3) = x_measure(3);
    x_tilde(4) = x_measure(4);
    
% Konstanten
    K = [ -0.1291    1.5139   -0.0655    0.1538]; %LQR
    drehmoment_soll =-K*x_tilde;
    

end

== matlab function furuta_model_mabx3/Control1/DiscreteStateSpaceMethods/LQR_aktiv ==
  data: x input; aktiv output
function aktiv = fcn(x)
% Konstanten
r_theta = 0.25*1.1; %[rad]
r_omega = 4*1.25; %[rad/s]

persistent einzugsbereich 
if isempty(einzugsbereich )
einzugsbereich = 0;
end
% Zustand
theta2 = x(2);
omega2 = x(4);

% Ausgang berechnen
if theta2^2/r_theta^2+omega2^2/r_omega^2 <= 1 
    einzugsbereich = 1;
end
if theta2<-pi/4||theta2>pi/4
    einzugsbereich = 0;
end
% Ausgang setzen
aktiv = einzugsbereich;
